simulink model "complementary_filter"  (R2022b)
settings: Solver=ode4  StartTime=TIME.Start  StopTime=TIME.Final  FixedStep=TIME.Ts  RelTol=1e-3
values from neighbouring files (symbols this model uses):
  C1 = 3 / tau    (= 7.5)    [Height_Filter.m]    (also in filter_simulation.m = 3)
  C2 = 2 * ws2 + 3 / tau^2    [Height_Filter.m]    (also in filter_simulation.m = 3.00000306683)
  C3 = 1 / tau^3    (= 15.625)    [Height_Filter.m]    (also in filter_simulation.m = 1)
  h_init = 0    [Height_Filter.m]
  vd_init = 0    [Height_Filter.m]
  ws2 = EARTH.g0 / EARTH.Req    [Height_Filter.m]    (also in filter_simulation.m = 1.53341296996e-06)
settings Model: Creator=jarry_goon  LastModifiedBy=jarry_goon

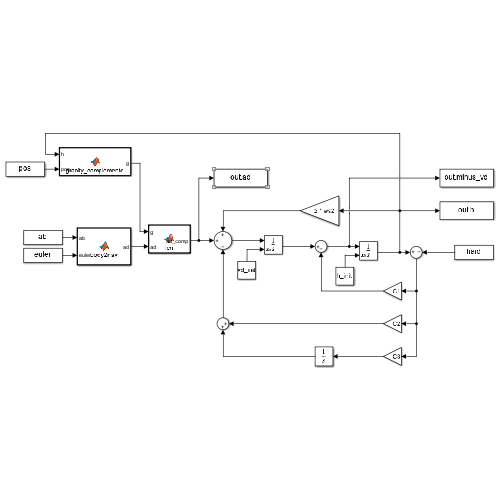
[thumbnail: Simulink's stored preview of the top-level diagram]
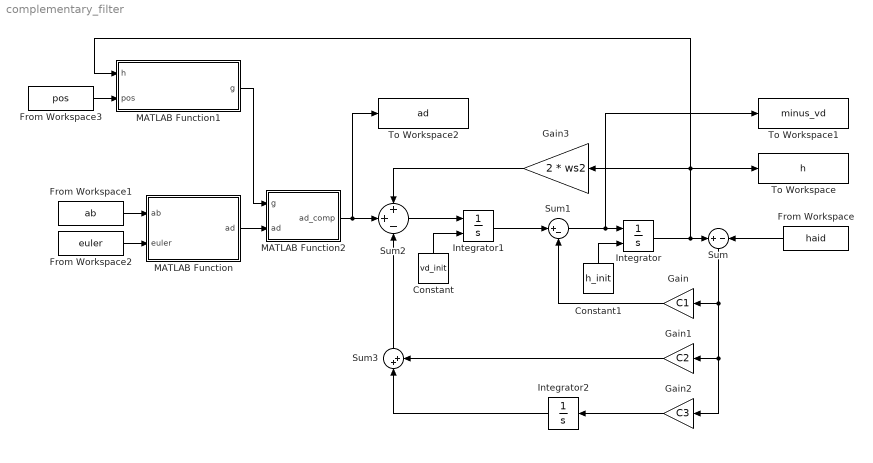
== system complementary_filter ==
  Constant : Constant  Value=vd_init
  Constant1 : Constant  Value=h_init
  From Workspace : FromWorkspace  VariableName=haid
  From Workspace1 : FromWorkspace  VariableName=ab
  From Workspace2 : FromWorkspace  VariableName=euler
  From Workspace3 : FromWorkspace  VariableName=pos
  Gain : Gain  Gain=C1
  Gain1 : Gain  Gain=C2
  Gain2 : Gain  Gain=C3
  Gain3 : Gain  Gain=2 * ws2
  Integrator : Integrator  InitialConditionSource=external
  Integrator1 : Integrator  InitialConditionSource=external
  Integrator2 : Integrator
  MATLAB Function : MATLAB Function  TreatAsAtomicUnit=on
  MATLAB Function1 : MATLAB Function  TreatAsAtomicUnit=on
  MATLAB Function2 : MATLAB Function  TreatAsAtomicUnit=on
  Sum : Sum  Inputs=+|-
  Sum1 : Sum  Inputs=|+-
  Sum2 : Sum  Inputs=++-
  Sum3 : Sum  Inputs=|++
  To Workspace : ToWorkspace  VariableName=h  SampleTime=-1
      settings: Save2DSignal=2-D array (concatenate along first dimension)
  To Workspace1 : ToWorkspace  VariableName=minus_vd  SampleTime=-1
      settings: Save2DSignal=2-D array (concatenate along first dimension)
  To Workspace2 : ToWorkspace  VariableName=ad  SampleTime=-1
      settings: Save2DSignal=2-D array (concatenate along first dimension)
  wires:
  Integrator/1 -> MATLAB Function1/1(h), Gain3/1, To Workspace/1, Sum/1
  Sum/1 -> Gain2/1, Gain1/1, Gain/1
  Sum1/1 -> To Workspace1/1, Integrator/1
  Gain/1 -> Sum1/2
  Integrator1/1 -> Sum1/1
  Sum2/1 -> Integrator1/1
  Gain1/1 -> Sum3/2
  Gain2/1 -> Integrator2/1
  Integrator2/1 -> Sum3/1
  Sum3/1 -> Sum2/3
  Gain3/1 -> Sum2/1
  Constant/1 -> Integrator1/2
  Constant1/1 -> Integrator/2
  From Workspace1/1 -> MATLAB Function/1(ab)
  From Workspace2/1 -> MATLAB Function/2(euler)
  From Workspace3/1 -> MATLAB Function1/2(pos)
  MATLAB Function/1(ad) -> MATLAB Function2/2(ad)
  MATLAB Function1/1(g) -> MATLAB Function2/1(g)
  MATLAB Function2/1(ad_comp) -> Sum2/2, To Workspace2/1
  From Workspace/1 -> Sum/2

== matlab function complementary_filter/MATLAB Function ==
  data: ab input; ad output; euler input
function ad = body2nav(ab, euler)

arguments
    ab (1, 3) double
    euler (1, 3) double
end

phi = euler(1); sin_phi = sin(phi); cos_phi = cos(phi);
the = euler(2); sin_the = sin(the); cos_the = cos(the);
psi = euler(3); sin_psi = sin(psi); cos_psi = cos(psi);

rx = [1         0          0;
      0         cos_phi    sin_phi;
      0        -sin_phi    cos_phi];

ry = [cos_the    0        -sin_the;
      0          1         0;
      sin_the    0         cos_the];

rz = [cos_psi    sin_psi    0;
     -sin_psi    cos_psi    0;
      0          0          1];

an = (rx * ry * rz)' * ab';

ad = an(3);

== matlab function complementary_filter/MATLAB Function2 ==
  data: g input; ad_comp output; ad input
function ad_comp = fcn(g, ad)

if ad == 0
    ad_comp = 0;
else
    ad_comp = -ad - g;
end

== matlab function complementary_filter/MATLAB Function1 ==
  data: h input; pos input; g output
function g = gracity_complemente(h, pos)

arguments
    h (1, 1) double
    pos (1, 2) double
end

e2 = 6.69437999014e-3;
Re = 6378137;
g0 = 9.780318;

sinL = sin(pos(1));
sin2L = sin(2 * pos(1));

R0 = Re * sqrt(1 - e2) / (1 - e2 * sinL^2);

g = g0 * (1 + 5.3024e-3 * sinL^2 - 5.9e-6 * sin2L^2);
g = g / (1 + h / R0)^2;
